simulink model "qbot2_sim_2020a"  (R2020a)
settings: Solver=FixedStepAuto  StartTime=0.0  StopTime=P.t_end  FixedStep=P.dt  RelTol=1e-3
InitFcn:
  | % load_qbot2_sim
StopFcn:
  | if (P.plotsim_flag)
  |     plot_sim(out, P)
  | end
settings Model: Creator=David L Olson  LastModifiedBy=divad

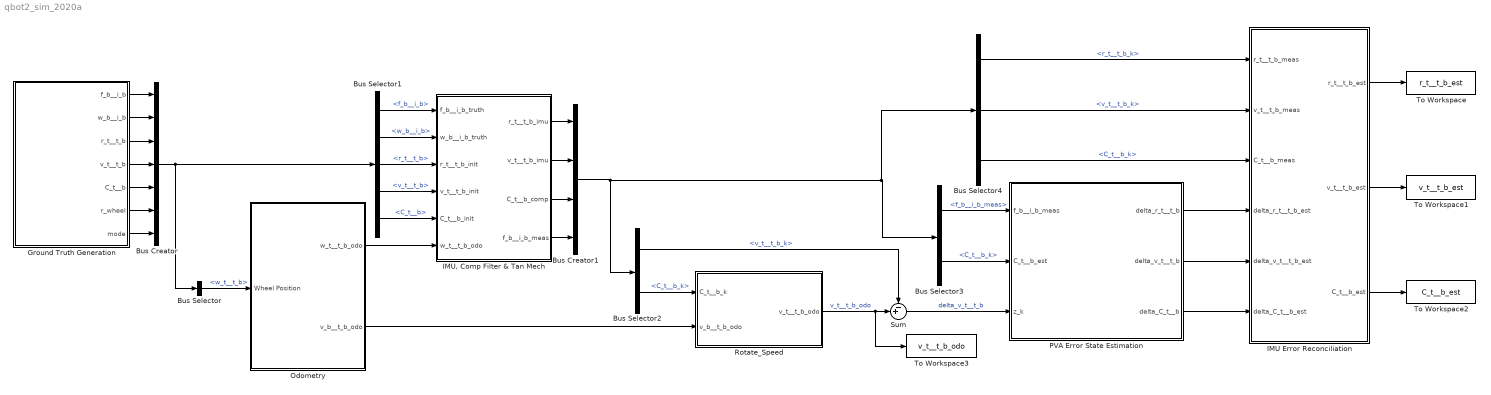
== system qbot2_sim_2020a ==
  Bus Creator : BusCreator  Inputs=7
  Bus Creator1 : BusCreator  Inputs=4
  Bus Selector : BusSelector  OutputSignals=w_t__t_b
  Bus Selector1 : BusSelector  OutputSignals=f_b__i_b,w_b__i_b,r_t__t_b,v_t__t_b,C_t__b
  Bus Selector2 : BusSelector  OutputSignals=v_t__t_b_k,C_t__b_k
  Bus Selector3 : BusSelector  OutputSignals=f_b__i_b_meas,C_t__b_k
  Bus Selector4 : BusSelector  OutputSignals=r_t__t_b_k,v_t__t_b_k,C_t__b_k
  Ground Truth Generation : Subsystem
  IMU Error Reconciliation : MATLAB Function  TreatAsAtomicUnit=on
  "IMU, Comp Filter & Tan Mech" : Subsystem
  Odometry : Subsystem
  PVA Error State Estimation : Subsystem
  Rotate_Speed : MATLAB Function  TreatAsAtomicUnit=on
  Sum : Sum  Inputs=-+|
  To Workspace : ToWorkspace  VariableName=r_t__t_b_est  SampleTime=-1
  To Workspace1 : ToWorkspace  VariableName=v_t__t_b_est  SampleTime=-1
  To Workspace2 : ToWorkspace  VariableName=C_t__b_est  SampleTime=-1
  To Workspace3 : ToWorkspace  VariableName=v_t__t_b_odo  SampleTime=-1
  wires:
  Ground Truth Generation/1(f_b__i_b) -> Bus Creator/1
  Ground Truth Generation/2(w_b__i_b) -> Bus Creator/2
  Ground Truth Generation/3(r_t__t_b) -> Bus Creator/3
  Ground Truth Generation/4(v_t__t_b) -> Bus Creator/4
  Ground Truth Generation/5(C_t__b) -> Bus Creator/5
  Bus Creator/1 -> Bus Selector1/1, Bus Selector/1
  Ground Truth Generation/6(r_wheel) -> Bus Creator/6
  Ground Truth Generation/7(mode) -> Bus Creator/7
  Bus Selector/1 -> Odometry/1(Wheel Position)  "<w_t__t_b>"
  Bus Selector1/1 -> "IMU, Comp Filter & Tan Mech"/1(f_b__i_b_truth)  "<f_b__i_b>"
  Bus Selector1/2 -> "IMU, Comp Filter & Tan Mech"/2(w_b__i_b_truth)  "<w_b__i_b>"
  Bus Selector1/3 -> "IMU, Comp Filter & Tan Mech"/3(r_t__t_b_init)  "<r_t__t_b>"
  Bus Selector1/4 -> "IMU, Comp Filter & Tan Mech"/4(v_t__t_b_init)  "<v_t__t_b>"
  Bus Selector1/5 -> "IMU, Comp Filter & Tan Mech"/5(C_t__b_init)  "<C_t__b>"
  Sum/1 -> PVA Error State Estimation/3(z_k)  "delta_v_t__t_b"
  Odometry/1(w_t__t_b_odo) -> "IMU, Comp Filter & Tan Mech"/6(w_t__t_b_odo)
  Odometry/2(v_b__t_b_odo) -> Rotate_Speed/2(v_b__t_b_odo)
  Rotate_Speed/1(v_t__t_b_odo) -> To Workspace3/1, Sum/2  "v_t__t_b_odo"
  "IMU, Comp Filter & Tan Mech"/1(r_t__t_b_imu) -> Bus Creator1/1
  "IMU, Comp Filter & Tan Mech"/2(v_t__t_b_imu) -> Bus Creator1/2
  "IMU, Comp Filter & Tan Mech"/3(C_t__b_comp) -> Bus Creator1/3
  "IMU, Comp Filter & Tan Mech"/4(f_b__i_b_meas) -> Bus Creator1/4
  Bus Creator1/1 -> Bus Selector4/1, Bus Selector3/1, Bus Selector2/1
  Bus Selector2/2 -> Rotate_Speed/1(C_t__b_k)  "<C_t__b_k>"
  Bus Selector2/1 -> Sum/1  "<v_t__t_b_k>"
  Bus Selector3/1 -> PVA Error State Estimation/1(f_b__i_b_meas)  "<f_b__i_b_meas>"
  Bus Selector3/2 -> PVA Error State Estimation/2(C_t__b_est)  "<C_t__b_k>"
  PVA Error State Estimation/1(delta_r_t__t_b) -> IMU Error Reconciliation/4(delta_r_t__t_b_est)
  PVA Error State Estimation/2(delta_v_t__t_b) -> IMU Error Reconciliation/5(delta_v_t__t_b_est)
  PVA Error State Estimation/3(delta_C_t__b) -> IMU Error Reconciliation/6(delta_C_t__b_est)
  Bus Selector4/1 -> IMU Error Reconciliation/1(r_t__t_b_meas)  "<r_t__t_b_k>"
  Bus Selector4/2 -> IMU Error Reconciliation/2(v_t__t_b_meas)  "<v_t__t_b_k>"
  Bus Selector4/3 -> IMU Error Reconciliation/3(C_t__b_meas)  "<C_t__b_k>"
  IMU Error Reconciliation/1(r_t__t_b_est) -> To Workspace/1
  IMU Error Reconciliation/3(C_t__b_est) -> To Workspace2/1
  IMU Error Reconciliation/2(v_t__t_b_est) -> To Workspace1/1

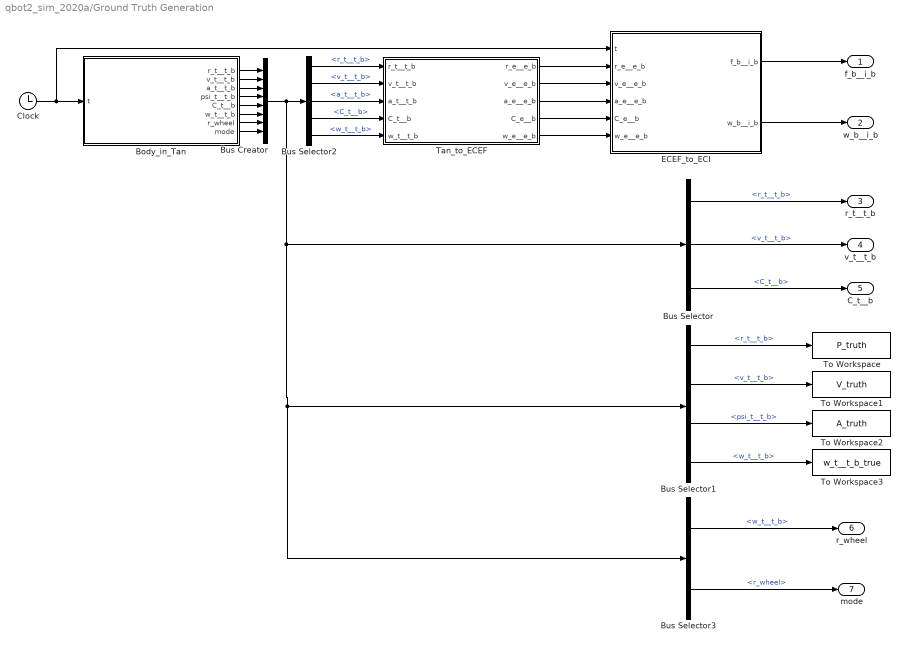
== system qbot2_sim_2020a/Ground Truth Generation ==
  Body_in_Tan : MATLAB Function  TreatAsAtomicUnit=on
  Bus Creator : BusCreator  Inputs=8
  Bus Selector : BusSelector  OutputSignals=r_t__t_b,v_t__t_b,C_t__b
  Bus Selector1 : BusSelector  OutputSignals=r_t__t_b,v_t__t_b,psi_t__t_b,w_t__t_b
  Bus Selector2 : BusSelector  OutputSignals=r_t__t_b,v_t__t_b,a_t__t_b,C_t__b,w_t__t_b
  Bus Selector3 : BusSelector  OutputSignals=w_t__t_b,r_wheel
  Clock : Clock
  ECEF_to_ECI : MATLAB Function  TreatAsAtomicUnit=on
  Tan_to_ECEF : MATLAB Function  TreatAsAtomicUnit=on
  To Workspace : ToWorkspace  VariableName=P_truth  SampleTime=-1
  To Workspace1 : ToWorkspace  VariableName=V_truth  SampleTime=-1
  To Workspace2 : ToWorkspace  VariableName=A_truth  SampleTime=-1
  To Workspace3 : ToWorkspace  VariableName=w_t__t_b_true  SampleTime=-1
  f_b__i_b : Outport
  w_b__i_b : Outport  Port=2
  r_t__t_b : Outport  Port=3
  v_t__t_b : Outport  Port=4
  C_t__b : Outport  Port=5
  r_wheel : Outport  Port=6
  mode : Outport  Port=7
  wires:
  Clock/1 -> Body_in_Tan/1(t), ECEF_to_ECI/1(t)
  Tan_to_ECEF/1(r_e__e_b) -> ECEF_to_ECI/2(r_e__e_b)
  Tan_to_ECEF/3(a_e__e_b) -> ECEF_to_ECI/4(a_e__e_b)
  Tan_to_ECEF/2(v_e__e_b) -> ECEF_to_ECI/3(v_e__e_b)
  Tan_to_ECEF/4(C_e__b) -> ECEF_to_ECI/5(C_e__b)
  Tan_to_ECEF/5(w_e__e_b) -> ECEF_to_ECI/6(w_e__e_b)
  ECEF_to_ECI/2(w_b__i_b) -> w_b__i_b/1
  ECEF_to_ECI/1(f_b__i_b) -> f_b__i_b/1
  Bus Selector/1 -> r_t__t_b/1  "<r_t__t_b>"
  Bus Selector/2 -> v_t__t_b/1  "<v_t__t_b>"
  Bus Selector/3 -> C_t__b/1  "<C_t__b>"
  Bus Selector2/5 -> Tan_to_ECEF/5(w_t__t_b)  "<w_t__t_b>"
  Bus Selector2/4 -> Tan_to_ECEF/4(C_t__b)  "<C_t__b>"
  Bus Selector2/3 -> Tan_to_ECEF/3(a_t__t_b)  "<a_t__t_b>"
  Bus Selector2/2 -> Tan_to_ECEF/2(v_t__t_b)  "<v_t__t_b>"
  Bus Selector2/1 -> Tan_to_ECEF/1(r_t__t_b)  "<r_t__t_b>"
  Bus Selector1/2 -> To Workspace1/1  "<v_t__t_b>"
  Bus Selector1/1 -> To Workspace/1  "<r_t__t_b>"
  Bus Selector1/3 -> To Workspace2/1  "<psi_t__t_b>"
  Bus Creator/1 -> Bus Selector/1, Bus Selector3/1, Bus Selector1/1, Bus Selector2/1
  Bus Selector3/1 -> r_wheel/1  "<w_t__t_b>"
  Bus Selector3/2 -> mode/1  "<r_wheel>"
  Body_in_Tan/1(r_t__t_b) -> Bus Creator/1
  Body_in_Tan/2(v_t__t_b) -> Bus Creator/2
  Body_in_Tan/3(a_t__t_b) -> Bus Creator/3
  Body_in_Tan/4(psi_t__t_b) -> Bus Creator/4
  Body_in_Tan/5(C_t__b) -> Bus Creator/5
  Body_in_Tan/6(w_t__t_b) -> Bus Creator/6
  Body_in_Tan/7(r_wheel) -> Bus Creator/7
  Body_in_Tan/8(mode) -> Bus Creator/8
  Bus Selector1/4 -> To Workspace3/1  "<w_t__t_b>"

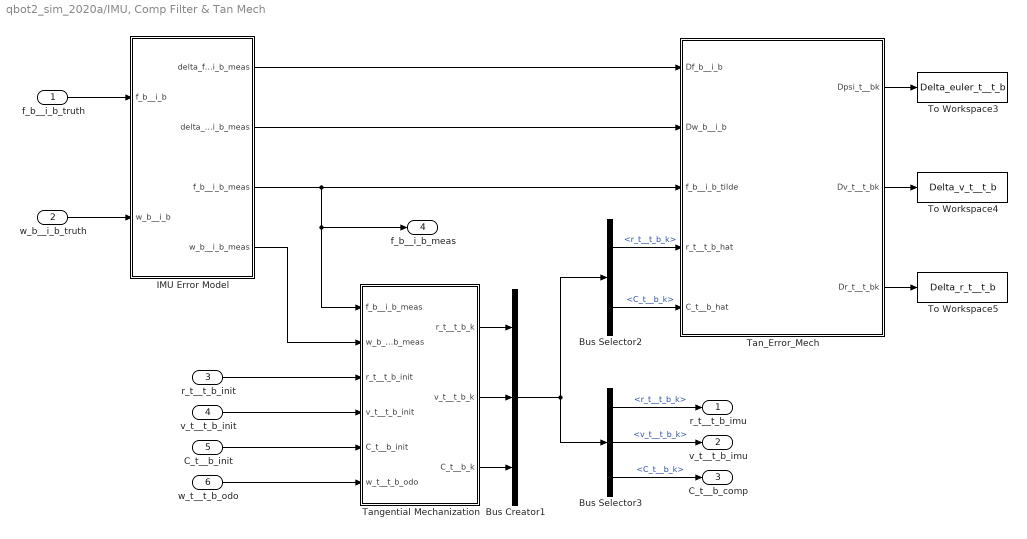
== system qbot2_sim_2020a/IMU, Comp Filter & Tan Mech ==
  f_b__i_b_truth : Inport
  w_b__i_b_truth : Inport  Port=2
  r_t__t_b_init : Inport  Port=3
  v_t__t_b_init : Inport  Port=4
  C_t__b_init : Inport  Port=5
  w_t__t_b_odo : Inport  Port=6
  Bus Creator1 : BusCreator  Inputs=3
  Bus Selector2 : BusSelector  OutputSignals=r_t__t_b_k,C_t__b_k
  Bus Selector3 : BusSelector  OutputSignals=r_t__t_b_k,v_t__t_b_k,C_t__b_k
  IMU Error Model : Subsystem
  Tan_Error_Mech : MATLAB Function  TreatAsAtomicUnit=on
  Tangential Mechanization : Subsystem
  To Workspace3 : ToWorkspace  VariableName=Delta_euler_t__t_b  SampleTime=-1
  To Workspace4 : ToWorkspace  VariableName=Delta_v_t__t_b  SampleTime=-1
  To Workspace5 : ToWorkspace  VariableName=Delta_r_t__t_b  SampleTime=-1
  r_t__t_b_imu : Outport
  v_t__t_b_imu : Outport  Port=2
  C_t__b_comp : Outport  Port=3
  f_b__i_b_meas : Outport  Port=4
  wires:
  f_b__i_b_truth/1 -> IMU Error Model/1(f_b__i_b)
  IMU Error Model/4(w_b__i_b_meas) -> Tangential Mechanization/2(w_b__i_b_meas)
  Tangential Mechanization/3(C_t__b_k) -> Bus Creator1/3
  IMU Error Model/1(delta_f_b__i_b_meas) -> Tan_Error_Mech/1(Df_b__i_b)
  IMU Error Model/3(f_b__i_b_meas) -> Tangential Mechanization/1(f_b__i_b_meas), f_b__i_b_meas/1, Tan_Error_Mech/3(f_b__i_b_tilde)
  w_b__i_b_truth/1 -> IMU Error Model/2(w_b__i_b)
  Tangential Mechanization/2(v_t__t_b_k) -> Bus Creator1/2
  IMU Error Model/2(delta_w_b__i_b_meas) -> Tan_Error_Mech/2(Dw_b__i_b)
  Tangential Mechanization/1(r_t__t_b_k) -> Bus Creator1/1
  Bus Selector2/2 -> Tan_Error_Mech/5(C_t__b_hat)  "<C_t__b_k>"
  C_t__b_init/1 -> Tangential Mechanization/5(C_t__b_init)
  v_t__t_b_init/1 -> Tangential Mechanization/4(v_t__t_b_init)
  Bus Creator1/1 -> Bus Selector2/1, Bus Selector3/1
  Bus Selector3/2 -> v_t__t_b_imu/1  "<v_t__t_b_k>"
  Bus Selector2/1 -> Tan_Error_Mech/4(r_t__t_b_hat)  "<r_t__t_b_k>"
  Bus Selector3/1 -> r_t__t_b_imu/1  "<r_t__t_b_k>"
  r_t__t_b_init/1 -> Tangential Mechanization/3(r_t__t_b_init)
  Tan_Error_Mech/3(Dr_t__t_bk) -> To Workspace5/1
  Tan_Error_Mech/1(Dpsi_t__bk) -> To Workspace3/1
  Tan_Error_Mech/2(Dv_t__t_bk) -> To Workspace4/1
  w_t__t_b_odo/1 -> Tangential Mechanization/6("w_t__t_b_odo ")
  Bus Selector3/3 -> C_t__b_comp/1  "<C_t__b_k>"

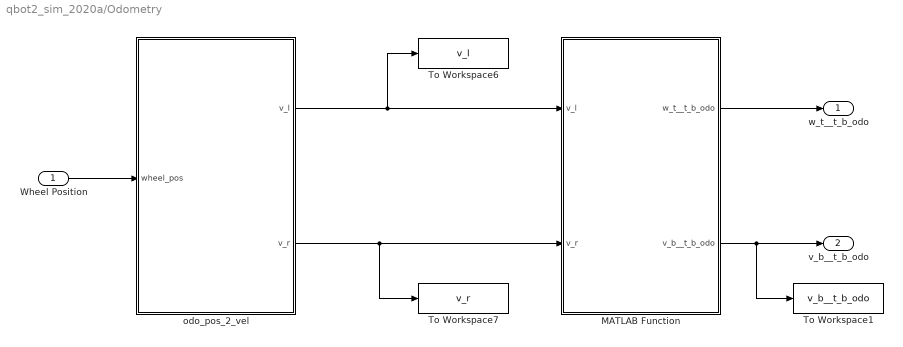
== system qbot2_sim_2020a/Odometry ==
  Wheel Position : Inport
  MATLAB Function : MATLAB Function  TreatAsAtomicUnit=on
  To Workspace1 : ToWorkspace  VariableName=v_b__t_b_odo  SampleTime=-1
  To Workspace6 : ToWorkspace  VariableName=v_l  SampleTime=-1
  To Workspace7 : ToWorkspace  VariableName=v_r  SampleTime=-1
  odo_pos_2_vel : MATLAB Function  TreatAsAtomicUnit=on
  w_t__t_b_odo : Outport
  v_b__t_b_odo : Outport  Port=2
  wires:
  Wheel Position/1 -> odo_pos_2_vel/1(wheel_pos)
  MATLAB Function/1(w_t__t_b_odo) -> w_t__t_b_odo/1
  odo_pos_2_vel/1(v_l) -> To Workspace6/1, MATLAB Function/1(v_l)
  odo_pos_2_vel/2(v_r) -> To Workspace7/1, MATLAB Function/2(v_r)
  MATLAB Function/2(v_b__t_b_odo) -> To Workspace1/1, v_b__t_b_odo/1

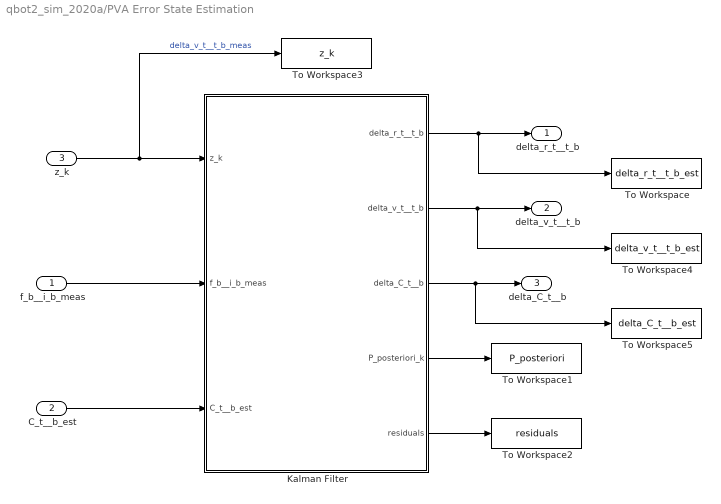
== system qbot2_sim_2020a/PVA Error State Estimation ==
  f_b__i_b_meas : Inport
  C_t__b_est : Inport  Port=2
  z_k : Inport  Port=3
  Kalman Filter : MATLAB Function  TreatAsAtomicUnit=on
  To Workspace : ToWorkspace  VariableName=delta_r_t__t_b_est  SampleTime=-1
  To Workspace1 : ToWorkspace  VariableName=P_posteriori  SampleTime=-1
  To Workspace2 : ToWorkspace  VariableName=residuals  SampleTime=-1
  To Workspace3 : ToWorkspace  VariableName=z_k  SampleTime=-1
  To Workspace4 : ToWorkspace  VariableName=delta_v_t__t_b_est  SampleTime=-1
  To Workspace5 : ToWorkspace  VariableName=delta_C_t__b_est  SampleTime=-1
  delta_r_t__t_b : Outport
  delta_v_t__t_b : Outport  Port=2
  delta_C_t__b : Outport  Port=3
  wires:
  Kalman Filter/4(P_posteriori_k) -> To Workspace1/1
  f_b__i_b_meas/1 -> Kalman Filter/2(f_b__i_b_meas)
  C_t__b_est/1 -> Kalman Filter/3(C_t__b_est)
  Kalman Filter/5(residuals) -> To Workspace2/1
  z_k/1 -> To Workspace3/1, Kalman Filter/1(z_k)  "delta_v_t__t_b_meas"
  Kalman Filter/1(delta_r_t__t_b) -> To Workspace/1, delta_r_t__t_b/1
  Kalman Filter/2(delta_v_t__t_b) -> To Workspace4/1, delta_v_t__t_b/1
  Kalman Filter/3(delta_C_t__b) -> To Workspace5/1, delta_C_t__b/1

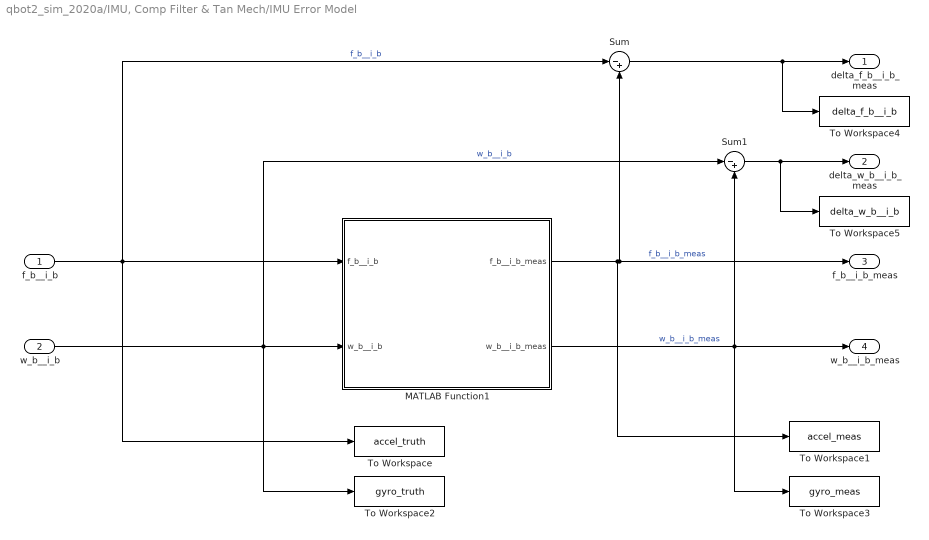
== system qbot2_sim_2020a/IMU, Comp Filter & Tan Mech/IMU Error Model ==
  f_b__i_b : Inport
  w_b__i_b : Inport  Port=2
  MATLAB Function1 : MATLAB Function  TreatAsAtomicUnit=on
  Sum : Sum  Inputs=|-+
  Sum1 : Sum  Inputs=|-+
  To Workspace : ToWorkspace  VariableName=accel_truth  SampleTime=-1
  To Workspace1 : ToWorkspace  VariableName=accel_meas  SampleTime=-1
  To Workspace2 : ToWorkspace  VariableName=gyro_truth  SampleTime=-1
  To Workspace3 : ToWorkspace  VariableName=gyro_meas  SampleTime=-1
  To Workspace4 : ToWorkspace  VariableName=delta_f_b__i_b  SampleTime=-1
  To Workspace5 : ToWorkspace  VariableName=delta_w_b__i_b  SampleTime=-1
  delta_f_b__i_b_meas : Outport
  delta_w_b__i_b_meas : Outport  Port=2
  f_b__i_b_meas : Outport  Port=3
  w_b__i_b_meas : Outport  Port=4
  wires:
  f_b__i_b/1 -> To Workspace/1, Sum/1, MATLAB Function1/1(f_b__i_b)  "f_b__i_b"
  w_b__i_b/1 -> Sum1/1, To Workspace2/1, MATLAB Function1/2(w_b__i_b)  "w_b__i_b"
  MATLAB Function1/1(f_b__i_b_meas) -> f_b__i_b_meas/1, Sum/2, To Workspace1/1  "f_b__i_b_meas"
  MATLAB Function1/2(w_b__i_b_meas) -> Sum1/2, w_b__i_b_meas/1, To Workspace3/1  "w_b__i_b_meas"
  Sum1/1 -> To Workspace5/1, delta_w_b__i_b_meas/1
  Sum/1 -> To Workspace4/1, delta_f_b__i_b_meas/1

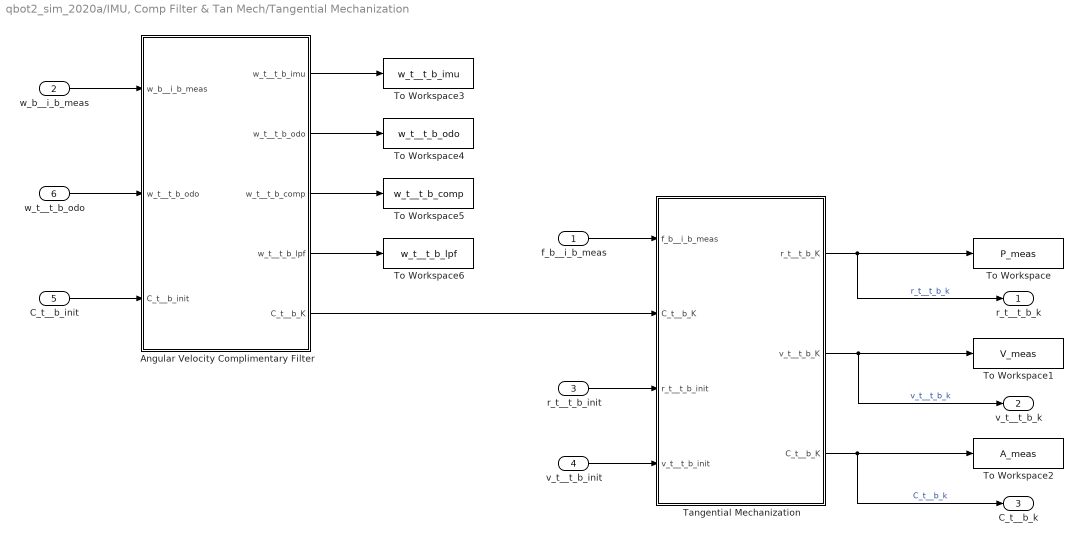
== system qbot2_sim_2020a/IMU, Comp Filter & Tan Mech/Tangential Mechanization ==
  f_b__i_b_meas : Inport
  w_b__i_b_meas : Inport  Port=2
  r_t__t_b_init : Inport  Port=3
  v_t__t_b_init : Inport  Port=4
  C_t__b_init : Inport  Port=5
  "w_t__t_b_odo " : Inport  Port=6
  Angular Velocity Complimentary Filter : MATLAB Function  TreatAsAtomicUnit=on
  Tangential Mechanization : MATLAB Function  TreatAsAtomicUnit=on
  To Workspace : ToWorkspace  VariableName=P_meas  SampleTime=-1
  To Workspace1 : ToWorkspace  VariableName=V_meas  SampleTime=-1
  To Workspace2 : ToWorkspace  VariableName=A_meas  SampleTime=-1
  To Workspace3 : ToWorkspace  VariableName=w_t__t_b_imu  SampleTime=-1
  To Workspace4 : ToWorkspace  VariableName=w_t__t_b_odo  SampleTime=-1
  To Workspace5 : ToWorkspace  VariableName=w_t__t_b_comp  SampleTime=-1
  To Workspace6 : ToWorkspace  VariableName=w_t__t_b_lpf  SampleTime=-1
  r_t__t_b_k : Outport
  v_t__t_b_k : Outport  Port=2
  C_t__b_k : Outport  Port=3
  wires:
  Tangential Mechanization/3(C_t__b_K) -> C_t__b_k/1, To Workspace2/1  "C_t__b_k"
  Tangential Mechanization/1(r_t__t_b_K) -> r_t__t_b_k/1, To Workspace/1  "r_t__t_b_k"
  Tangential Mechanization/2(v_t__t_b_K) -> v_t__t_b_k/1, To Workspace1/1  "v_t__t_b_k"
  f_b__i_b_meas/1 -> Tangential Mechanization/1(f_b__i_b_meas)
  r_t__t_b_init/1 -> Tangential Mechanization/3(r_t__t_b_init)
  v_t__t_b_init/1 -> Tangential Mechanization/4(v_t__t_b_init)
  w_b__i_b_meas/1 -> Angular Velocity Complimentary Filter/1(w_b__i_b_meas)
  C_t__b_init/1 -> Angular Velocity Complimentary Filter/3(C_t__b_init)
  "w_t__t_b_odo "/1 -> Angular Velocity Complimentary Filter/2("w_t__t_b_odo ")
  Angular Velocity Complimentary Filter/5(C_t__b_K) -> Tangential Mechanization/2("C_t__b_K ")
  Angular Velocity Complimentary Filter/1(w_t__t_b_imu) -> To Workspace3/1
  Angular Velocity Complimentary Filter/2(w_t__t_b_odo) -> To Workspace4/1
  Angular Velocity Complimentary Filter/3(w_t__t_b_comp) -> To Workspace5/1
  Angular Velocity Complimentary Filter/4(w_t__t_b_lpf) -> To Workspace6/1

== matlab function qbot2_sim_2020a/IMU Error Reconciliation ==
  data: r_t__t_b_meas input; r_t__t_b_est output; v_t__t_b_meas input; C_t__b_meas input; v_t__t_b_est output; C_t__b_est output; delta_r_t__t_b_est input; delta_v_t__t_b_est input; delta_C_t__b_est input
function [r_t__t_b_est, v_t__t_b_est, C_t__b_est] = ...
    imu_error_reconcile(r_t__t_b_meas, v_t__t_b_meas, C_t__b_meas, ...
                        delta_r_t__t_b_est, delta_v_t__t_b_est, delta_C_t__b_est)

% Reconclie Position
r_t__t_b_est = r_t__t_b_meas - delta_r_t__t_b_est;

% Reconcile Velocity
v_t__t_b_est = v_t__t_b_meas - delta_v_t__t_b_est;

% Reconclie Attitude
C_t__b_est = C_t__b_meas * delta_C_t__b_est;

== matlab function qbot2_sim_2020a/PVA Error State Estimation/Kalman Filter ==
  data: delta_r_t__t_b output; delta_v_t__t_b output; delta_C_t__b output; z_k input; f_b__i_b_meas input; C_t__b_est input; P parameter; P_posteriori_k output; residuals output
function [delta_r_t__t_b, delta_v_t__t_b, delta_C_t__b, P_posteriori_k, residuals] = ...
              IMU_Error_State_Estimation(z_k, f_b__i_b_meas, C_t__b_est, P)
%% IMU Error State Estimation Function
% Recieves error measurements from the difference between odometry and the
% IMU, and provides estimates of that error.  

persistent x_posteriori_k_1 P_posteriori_k_1 A Q_bar 

dt = P.dt;

% Normalize C_t__b_est
C_t__b_est = q2dcm(dcm2q(C_t__b_est));

%% Kalman Filter Prediction Steps

%**************************************************************************
% For first instance only
if (isempty(x_posteriori_k_1))
    
% Set Initial Values for x and P___________________________________________
    x_0 = zeros(15,1);
    P_0 = diag(1000 * [P.gyro.sigma_ARW.^2; ...
                      P.accel.sigma_VRW.^2; ...
                     (P.accel.sigma_VRW * dt).^2; ...
                      P.accel.BI.sigma_n.^2; ...
                      P.gyro.BI.sigma_n.^2]);
    x_posteriori_k_1 = zeros(15,1);
    P_posteriori_k_1 = eye(15);
    
% Build the Contiuous Time Model___________________________________________
    A = zeros(15, 15);
    
    % Values that vary with time
    f_b__i_b_est = f_b__i_b_meas;
    
    % Compute A - Fifth Row
    A(13:15, 13:15) = -eye(3) ./ P.gyro.BI.correlation_time;
    
    % Compute A - Fourth Row
    A(10:12, 10:12) = -eye(3) ./ P.accel.BI.correlation_time;
    
    % Compute A - Third Row
    A(7:9, 4:6) = eye(3);
    
    % Compute A - Second Row
    A(4:6, 1:3) = -vec2ss(C_t__b_est * f_b__i_b_est);
    A(4:6, 4:6) = -2 .* P.Ohm_t__i_e;
    A(4:6, 10:12) = -C_t__b_est;

    % Compute the monstrosity A(4:6, 7:9) a.k.a. A_23
    r_e__e_b_hat = P.r_e__e_t; % initial position is always the origin
    [L_b_hat, ~, ~] = xyz2llh(r_e__e_b_hat, P);
    g_0 = Somigliana(L_b_hat, P);
    r_e__e_S = Geo_Radius(L_b_hat, P);
    A(4:6, 7:9) = P.C_e__t' * ((2 * g_0 * r_e__e_b_hat) / (r_e__e_S * norm(r_e__e_b_hat)^2)) * r_e__e_b_hat' * P.C_e__t;
    
    % Compute A - First Row
    A(1:3, 1:3) = -P.Ohm_t__i_e;
    A(1:3, 13:15) = -C_t__b_est;
    
% Define Q_bar_____________________________________________________________
    Q_vec = [P.gyro.sigma_ARW.^2;   ...       % Attitude Process Noise rad/s
             P.accel.sigma_VRW.^2;  ...       % Velocity Process Noise m/s
             zeros(3,1);         ...          % Position Process Noise
             P.accel.BI.sigma_n.^2; ...       % Accel Bias Instability Process Noise m/s
             P.gyro.BI.sigma_n.^2];           % Gyro  Bias Instability Process Noise rad/s
     
    % Allow for a margin of error for tuning     
    Q_fudge_factor = 1;
    
    % Set Q
    Q_bar = diag(Q_fudge_factor .* Q_vec');
    
% Discritize the Continuous Time Model_____________________________________
    F = eye(15) + A*dt;
    Q = (1/2) * ((F*Q_bar*F') + Q_bar) * dt;
    
% Compute first prediction_________________________________________________
    x_priori_k = F * x_0;
    P_priori_k = (F * P_0 * F') + Q;
    
%**************************************************************************
% All other instances: State Prediction  
else
    
% Re-compute the time varying arguements of A______________________________
    
    % Values that vary with time
    f_b__i_b_est = f_b__i_b_meas;

    % Compute A - Second Row
    A(4:6, 1:3) = -vec2ss(C_t__b_est * f_b__i_b_est);
    A(4:6, 10:12) = -C_t__b_est;
    
    % Compute A - First Row
    A(1:3, 13:15) = -C_t__b_est;
    
% Discritize the Continuous Time Model_____________________________________
    F = eye(15) + A*dt;
    Q = (1/2) * ((F*Q_bar*F') + Q_bar) * dt;
    
    % Compute prediction step
    x_priori_k = (F * x_posteriori_k_1);
    P_priori_k = (F * P_posteriori_k_1 * F') + Q;
    
    % Symmetrisize P
    P_priori_k = (P_priori_k + P_priori_k') / 2;
    
end

%% Kalman Filter Measurement Update Steps
%**************************************************************************

% Set H Matrix - Velocity Aiding Only
H = [vec2ss(x_priori_k(4:6)), eye(3), zeros(3,9)]; % H = [(v_t__t_b,x), I_3, 0_3]

% Build R for odometry
var_v_b__t_b = [(P.sigma_odo_d / P.dt)^2; ...  % Variance of Speed in {b} frame
                 0.005^2; ...                  % Assumed Variance of body frame {y} vel, Nonholomonic Constraints
                 0.005^2];                     % Assumed Variance of body frame {z} vel, Nonholomonic Constraints

% Rotate Noise in {b} frame into the {t} frame
R_vec = C_t__b_est * var_v_b__t_b;

% Allow for Margin of Error
R_fudge_factor = 1.5;

% Set R
R = diag(R_fudge_factor .* R_vec);

% Kalman Gain Computation
K = (P_priori_k * H') / (H * P_priori_k * H' + R);

% compute residuals
residuals = z_k - H*x_priori_k;

% A Posteriori State and Covariance Update
x_posteriori_k = x_priori_k + K*(z_k - H*x_priori_k);
P_posteriori_k = (eye(15) - K*H) * P_priori_k;

%Symmetrisize P
P_posteriori_k = (P_posteriori_k + P_posteriori_k') / 2;

%% Pick-off State Estimates for Function Output

% State Estimates (AVP -> PVA)
delta_x_t__t_b_est = ...
           [x_posteriori_k(7:9); x_posteriori_k(4:6); x_posteriori_k(1:3)];

% Pull Off Position, Velocity, and Attitude Error Separately
delta_r_t__t_b = delta_x_t__t_b_est(1:3);
delta_v_t__t_b = delta_x_t__t_b_est(4:6);
delta_k_t__t_b = delta_x_t__t_b_est(7:9);

% Create and Normalize delta_C_t__b
delta_C_t__b = k2dcm(delta_k_t__t_b);
delta_C_t__b = q2dcm(dcm2q(delta_C_t__b));
       
%% Save State Estimates for Next Loop

x_posteriori_k_1 = x_posteriori_k;
P_posteriori_k_1 = P_posteriori_k;

end

== matlab function qbot2_sim_2020a/Odometry/odo_pos_2_vel ==
  data: wheel_pos input; v_l output; v_r output; P parameter
%% Odometry True Position to Noisy Wheel Velocities
function [v_l, v_r]= pos2vel(wheel_pos, P)
                                                     
% Initialize Inital Conditions
persistent d_l_k_1 d_r_k_1

if (isempty(d_l_k_1))
    d_l_k_1 = 0;
    d_r_k_1 = 0;
end

% ISolate current wheel positions
d_l_k = wheel_pos(1,:);
d_r_k = wheel_pos(2,:);

% Build randn quantities from etrinsic functions
coder.extrinsic('randn');

% Preallocate Memory
randn1 = 0;
randn2 = 0;

% Build the randn variables
randn1 = randn;
randn2 = randn;

% Add Noise to Measurements if desired
if (P.odo_error_flag == true)
    d_l_k = d_l_k + P.sigma_odo_d * randn1;
    d_r_k = d_r_k + P.sigma_odo_d * randn2;
end

% Take this psuedo non-casual derivative
v_l = (d_l_k - d_l_k_1) / P.dt;
v_r = (d_r_k - d_r_k_1) / P.dt;

% Set the Current Values as the Previous Values
d_l_k_1 = d_l_k;
d_r_k_1 = d_r_k;

== matlab function qbot2_sim_2020a/IMU, Comp Filter & Tan Mech/Tangential Mechanization/Angular Velocity Complimentary Filter ==
  data: w_b__i_b_meas input; w_t__t_b_imu output; w_t__t_b_odo input; C_t__b_init input; w_t__t_b_odo output; w_t__t_b_comp output; w_t__t_b_lpf output; C_t__b_K output; P parameter
function [w_t__t_b_imu, w_t__t_b_odo, w_t__t_b_comp, w_t__t_b_lpf, C_t__b_K] = ...
          complimentary_filter(w_b__i_b_meas, w_t__t_b_odo, C_t__b_init, P)

% This block implments a complimentary filter between z-gyro measurements
% and odometry angular veocity measurements and then provides a corrected
% version of C_t__b_k

persistent C_t__b_K_1 delta_w_t__t_b_k_1 delta_w_t__t_b_lpf_k_1

% Initialize on First Time Step
if (isempty(C_t__b_K_1))
    
    % Use "truth" to initialize on first time step
    C_t__b_K   = C_t__b_init;
    
    % Store current values as old values for next iteration
    C_t__b_K_1   = C_t__b_K;

    % Set Up Complimentary Filter Values
    delta_w_t__t_b_k_1 = zeros(3,1);
    delta_w_t__t_b_lpf_k_1 = zeros(3,1);
    
    % Return Other Output Values
    w_t__t_b_imu = C_t__b_K_1*w_b__i_b_meas - P.C_e__t'*P.w_i__i_e;
    w_t__t_b_comp = w_t__t_b_imu;
    w_t__t_b_lpf = w_t__t_b_imu;
    
%% For all other time steps
else
    
    % Employ Complimentary Filter__________________________________________
    if (P.use_comp_filter == true)
        
        % Calculate w_t__t_b_imu
        w_t__t_b_imu = C_t__b_K_1*w_b__i_b_meas - P.C_e__t'*P.w_i__i_e;
        
        % Take the differene between the odo and imu measurements
        delta_w_t__t_b = w_t__t_b_odo - w_t__t_b_imu;
        
        % Pass the w error through the Low Pass Filter (LPF)
        w_t__t_b_lpf = -P.lpf_den_1 .* delta_w_t__t_b_lpf_k_1 + ...
                        P.lpf_num_1 .* delta_w_t__t_b + ...
                        P.lpf_num_2 .* delta_w_t__t_b_k_1;
        
        % Sum up the LPF'd error and IMU meas
        w_t__t_b_comp = w_t__t_b_imu + w_t__t_b_lpf;
        
        % Catch for when w_t__t_b is super super small
        if (norm(w_t__t_b_comp) < (5 * eps))
            C_t__b_K = C_t__b_K_1;
        else
            C_t__b_K = Rodrigues_k(w_t__t_b_comp * P.dt) * C_t__b_K_1;
        end
    
    % If not using Complimentary Filter____________________________________
    else
        
        % Calculate w_t__t_b_imu
        w_t__t_b_imu = C_t__b_K_1*w_b__i_b_meas - P.C_e__t'*P.w_i__i_e;
        
        % Catch for when w_t__t_b is super super small
        if (norm(w_t__t_b_imu) < (5 * eps))
            C_t__b_K = C_t__b_K_1;
        else
            C_t__b_K = Rodrigues_k(w_t__t_b_imu * P.dt) * C_t__b_K_1;
        end
        
        % Return zeros for comp filter variables
        w_t__t_b_comp = zeros(3,1);
        w_t__t_b_lpf = zeros(3,1);
        delta_w_t__t_b = zeros(3,1);
        delta_w_t__t_b_k_1 = zeros(3,1);
        delta_w_t__t_b_lpf_k_1 = zeros(3,1);
        
    end
    
    % Normalize C_t__b_K___________________________________________________
    C_t__b_K = q2dcm(dcm2q(C_t__b_K));
    
    
% Store New Value as the Old_______________________________________________
C_t__b_K_1 = C_t__b_K;
delta_w_t__t_b_k_1 = delta_w_t__t_b;
delta_w_t__t_b_lpf_k_1 = w_t__t_b_lpf;

end

== matlab function qbot2_sim_2020a/Rotate_Speed ==
  data: C_t__b_k input; v_t__t_b_odo output; v_b__t_b_odo input
function v_t__t_b_odo = rotate_speed(C_t__b_k, v_b__t_b_odo)

% Rotate Speed in the body frame into the {t} frame
v_t__t_b_odo = C_t__b_k * v_b__t_b_odo;

== matlab function qbot2_sim_2020a/Ground Truth Generation/Body_in_Tan ==
  data: r_t__t_b output; v_t__t_b output; a_t__t_b output; psi_t__t_b output; C_t__b output; w_t__t_b output; t input; P parameter; r_wheel output; mode output
function [r_t__t_b, v_t__t_b, a_t__t_b, psi_t__t_b, C_t__b, w_t__t_b, r_wheel, mode] = ...
                                           Body_in_Tan(t, P)
                                       
%% QBOT2_TAN_GROUND_TRUTH_GEN Generates the motion of the body of the Qbot2
%wrt to the tangential frame.  

% Creating figure eight loop pattern for Qbot2.  The motion is unrealistic
% for the robot itself, however for now this verify all equations have been
% implemented correctly in all 3 dimensions.  

persistent k

% Initialize k on first run
if (isempty(k))
    k = 1;
end

% Pull Motion Plan Values from P structure
r_t__t_b = P.r_t__t_b(:,k);
v_t__t_b = P.v_t__t_b(:,k);
a_t__t_b = P.a_t__t_b(:,k);
psi_t__t_b = [0; 0; P.psi_t__t_b(k)];
C_t__b = rotate_z(psi_t__t_b(3));
w_t__t_b = P.w_t__t_b(:,k);
r_wheel = P.r_wheel(:,k);
mode = P.mode(k);

% Normalize C_t__b
C_t__b = q2dcm(dcm2q(C_t__b));

% Update k
k = k + 1;

end

== matlab function qbot2_sim_2020a/IMU, Comp Filter & Tan Mech/Tangential Mechanization/Tangential Mechanization ==
  data: f_b__i_b_meas input; C_t__b_K input; r_t__t_b_init input; v_t__t_b_init input; r_t__t_b_K output; P parameter; v_t__t_b_K output; C_t__b_K output
function [r_t__t_b_K, v_t__t_b_K, C_t__b_K] = Tan_Mech(f_b__i_b_meas, C_t__b_K, r_t__t_b_init, v_t__t_b_init, P)

%% Tan_Mech
% Provides tangential mechanization for kinematic states position, velocity
% and attitude (PVA).  It does this solely based on accel and gyro
% measurements, which come from the IMU block.  The first time step is
% initialized from the ground truth block.  

persistent r_t__t_b_K_1 v_t__t_b_K_1 g_t__b

% Initialize on First Time Step
if (isempty(r_t__t_b_K_1))
    
    % Use "truth" to initialize on first time step
    r_t__t_b_K = r_t__t_b_init;
    v_t__t_b_K = v_t__t_b_init;
    
    % Store current values as old values for next iteration
    r_t__t_b_K_1 = r_t__t_b_K;
    v_t__t_b_K_1 = v_t__t_b_K;
    
    % Calculate and store the vector g_t__b
    r_e__e_b = P.r_e__e_t + P.C_e__t*r_t__t_b_init;         % Compute r_e__e_b
    [L_b, lambda_b, h_b] = xyz2llh(r_e__e_b, P);            % Compute the lat, lon, and height
    g_n__b = [0; 0; gravity(L_b, h_b, P)];                  % Compute the acceleration due to gravity
    C_e__n = Lat_Lon_2C_e__n(L_b, lambda_b);                % Compute C_e__n
    g_e__b = C_e__n * g_n__b;                               % Compute the gravity of the body in the {e} frame
    g_t__b = P.C_e__t' * g_e__b;                            % Compute the gravity of the body in the {t} frame 
    
% Every Other Time Step____________________________________________________
else
    
    % f_t__i_b Specific Force Update
    f_t__i_b = C_t__b_K * f_b__i_b_meas;
    
    % a_t__t_b Acceleration Vector Update
    
    a_t__t_b = f_t__i_b + g_t__b - 2*P.Ohm_t__i_e*v_t__t_b_K_1;
    
    % v_t__t_b Velocity Vector Update
    v_t__t_b_K = v_t__t_b_K_1 + a_t__t_b*P.dt;
    
    % r_t__t_b Position Vector Update
    r_t__t_b_K = r_t__t_b_K_1 + v_t__t_b_K_1*P.dt + a_t__t_b*((P.dt^2)/2);
    
    % Store new PVA as old PVA
    r_t__t_b_K_1 = r_t__t_b_K;
    v_t__t_b_K_1 = v_t__t_b_K;
    
end

== matlab function qbot2_sim_2020a/Ground Truth Generation/Tan_to_ECEF ==
  data: r_t__t_b input; v_t__t_b input; a_t__t_b input; C_t__b input; w_t__t_b input; r_e__e_b output; v_e__e_b output; a_e__e_b output; C_e__b output; w_e__e_b output; P parameter
function [r_e__e_b, v_e__e_b, a_e__e_b, C_e__b, w_e__e_b] = ...
             Tan_to_ECEF(r_t__t_b, v_t__t_b, a_t__t_b, C_t__b, w_t__t_b, P)
         
%% Tan_to_ECEF 
% Transfroms motion in the {t} frame into the {e} frame.  The 'P' structure
% contains data relevant to making the {t}->{e} transforms specifically to
% my house in Minot ND.  (1124 9th St NW, Minot ND 58703)

% Position of the {b} frame wrt the {e} frame resolved in {e} (m)
r_e__e_b = P.r_e__e_t + P.C_e__t*r_t__t_b;

% Velocity of the {b} frame wrt the {e} frame resolved in {e} (m/s)
v_e__e_b = P.C_e__t*v_t__t_b;
       
% Acceleration of the b-frame wrt the e-frame resolved in {e} (m/s^2)
a_e__e_b = P.C_e__t*a_t__t_b;
        
%Attitude of the {b} frame wrt the {e} frame (unitless)
C_e__b = P.C_e__t*C_t__b;         

% Normalize C_e__b
C_e__b = q2dcm(dcm2q(C_e__b));

% Angular velocity of the {b} frame wrt the {e} frame resolved in {e} (rad/s)
w_e__e_b = P.C_e__t*w_t__t_b;

== matlab function qbot2_sim_2020a/Ground Truth Generation/ECEF_to_ECI ==
  data: t input; f_b__i_b output; r_e__e_b input; v_e__e_b input; a_e__e_b input; C_e__b input; w_e__e_b input; w_b__i_b output; P parameter
function [f_b__i_b, w_b__i_b] = ...
          ECEF_to_ECI(t, r_e__e_b, v_e__e_b, a_e__e_b, C_e__b, w_e__e_b, P)

%% ECEF to ECI
% Transforms motion from the ECEF frame to the ECI frame
% This assumes the simulation always starts at 0000z

% Calculate g_n__b only once, since area of travel is so small
persistent g_e__b

if (isempty(g_e__b))
    [L_b, lambda_b, h_b] = xyz2llh(r_e__e_b, P);
    g_n__b = [0; 0; gravity(L_b, h_b, P)];
    C_e__n = Lat_Lon_2C_e__n(L_b, lambda_b);
    g_e__b = C_e__n * g_n__b;
end

% Generate earth's rotation from {i} frame to {e} frame
theta_ie = P.w_ie * t + 0;

C_i__e = [cos(theta_ie), -sin(theta_ie), 0; ...
          sin(theta_ie),  cos(theta_ie), 0; ...
          0,              0,             1];    
      
% Position of {b} frame wrt {t} frame resolved in {i} frame (m)
r_i__i_b = C_i__e*r_e__e_b;

% Velocity of {b} frame wrt {i} frame resolved in {i} frame (m/s)
v_i__i_b = C_i__e*v_e__e_b + P.Ohm_i__i_e*C_i__e*r_e__e_b;

% Acceleration of {b} frame wrt {i} frame resolved in {i} frame (m/s^2)
a_i__i_b = C_i__e*a_e__e_b + 2*P.Ohm_i__i_e*C_i__e*v_e__e_b + ...
                                 P.Ohm_i__i_e*P.Ohm_i__i_e*C_i__e*r_e__e_b;
                                       
% Attitude of {b} frame wrt to {i} frame
C_i__b = C_i__e*C_e__b;

% Normalize C_i__b
C_i__b = q2dcm(dcm2q(C_i__b));

% Angular Velocity: Ideal Gyro Measurements
w_b__i_b = C_i__b' * (P.w_i__i_e + C_i__e*w_e__e_b);

% Specific Force: Ideal Accel Measurements
f_b__i_b = C_i__b' * (a_i__i_b - C_i__e*g_e__b - ...
                                       P.Ohm_i__i_e*P.Ohm_i__i_e*r_i__i_b);

== matlab function qbot2_sim_2020a/IMU, Comp Filter & Tan Mech/IMU Error Model/MATLAB Function1 ==
  data: f_b__i_b input; f_b__i_b_meas output; w_b__i_b input; w_b__i_b_meas output; P parameter
function [f_b__i_b_meas, w_b__i_b_meas] = IMU(f_b__i_b, w_b__i_b, P)
% IMU models the IMU error characteristics, taking truth as the input and
% outputs measurements that are subject to errors.  These errors stem from
% data obtained from the VN200 used for hardware implementation.  

%% Function Initializatoin

persistent b_g_BI b_a_BI

if isempty(b_g_BI)
    b_g_BI = [0; 0; 0];
    b_a_BI = [0; 0; 0];
end

%% Define P

%  General P
dt = P.dt;
Fs = P.Fs;
I3 = eye(3);

% Gyro Related Terms
b_g_BI_sigma_n = P.gyro.BI.sigma_n;  % Bias - White Noise driving the Bias Instability 1-sigma (rad/s)

tau_g        = P.gyro.BI.correlation_time;  % Correlation time for the bias instability (sec)
b_g_FB       = P.gyro.b_g_FB;               % Bias - Fixed Bias term (rad/s)

sigma_ARW   = P.gyro.sigma_ARW;             % Standard deviation of white noise due to ARW (rad/s)
M_g         = P.gyro.M_g;                   % The combined Gyro Misalignment/Scale-Factor matrix
G_g         = P.gyro.G_g;                   % The gyro G-sensitivity matrix (rad/sec/g)

 % Accel related terms   
b_a_BI_sigma_n = P.accel.BI.sigma_n;        % Bias - White noise driving the Bias Instability 1-sigma (m/s^2)

tau_a        = P.accel.BI.correlation_time; % Correlation time for the bias instability (sec)
b_a_FB       = P.accel.b_a_FB;              % Bias - Fixed Bias term (m/s^2)

sigma_VRW   = P.accel.sigma_VRW;            % Standard deviation of white noise due to VRW (m/s^2)
M_a         = P.accel.M_a;                  % The combined Gyro Misalignment/Scale-Factor matrix    

% Build randn quantities from etrinsic functions
coder.extrinsic('randn');

% Preallocate Memory
randn1 = zeros(3,1);
randn2 = zeros(3,1);
randn3 = zeros(3,1);
randn4 = zeros(3,1);

% Build the randn variables
randn1 = randn(3,1);
randn2 = randn(3,1);
randn3 = randn(3,1);
randn4 = randn(3,1);

%++++++++++++++++++++++++++++++++++++++++++++++++++++++++++++++++++++++++++
% Gyro Model:
%++++++++++++++++++++++++++++++++++++++++++++++++++++++++++++++++++++++++++

% Bias terms
b_g_BS = P.gyro.b_g_BS;                                        % Bias - Bias Stability Bias term (rad/s)
b_g_BI = exp(-dt/tau_g) * b_g_BI + randn1.*b_g_BI_sigma_n; % Bias - Markov Bias Instability Bias term (rad/s)
b_g = b_g_BI + b_g_FB + b_g_BS;                                % All three bias terms (rad/s)

% Noise terms
w_g = sigma_ARW .* randn2;                                 % Gyro noise (rad/sec)

% Including all of the error terms
w_b__i_b_meas = b_g + (I3 + M_g) * w_b__i_b + G_g * f_b__i_b + w_g;

%++++++++++++++++++++++++++++++++++++++++++++++++++++++++++++++++++++++++++
% Accelerometer Model
%++++++++++++++++++++++++++++++++++++++++++++++++++++++++++++++++++++++++++

% Bias terms
b_a_BS = P.accel.b_a_BS;                                       % Bias - Bias Stability Bias term (m/s^2)
b_a_BI = exp(-dt/tau_a) * b_a_BI + randn3.*b_a_BI_sigma_n; % Bias - Markov Bias Instability Bias term (m/s^2)
b_a = b_a_BI + b_a_FB + b_a_BS;                                % All three bias terms (m/s^2)

% Noise terms
w_a = sigma_VRW .* randn4;                                 % Accelerometer noise (in m/s^2)

% Including all of the error terms
f_b__i_b_meas = b_a + (I3 + M_a) * f_b__i_b + w_a;

== matlab function qbot2_sim_2020a/IMU, Comp Filter & Tan Mech/Tan_Error_Mech ==
  data: Df_b__i_b input; Dpsi_t__bk output; Dw_b__i_b input; f_b__i_b_tilde input; r_t__t_b_hat input; C_t__b_hat input; Dv_t__t_bk output; Dr_t__t_bk output; P parameter
function [Dpsi_t__bk, Dv_t__t_bk, Dr_t__t_bk] = Tan_Error_mech(Df_b__i_b, Dw_b__i_b, f_b__i_b_tilde, r_t__t_b_hat, C_t__b_hat, P)
%#codegen
% FUNCTION DESCRIPTION:
%   Implements the Tangential Frame Error-Mechanization
%
% INPUTS:
%   Df_b__i_b       = Error in Current Accel measurements (m/s^2)
%   Dw_b__i_b       = Error in Current gyro measurements (rad/s)
%   f_b__i_b_tilde  = Current Accel measurements (m/s^2)
%   r_t__t_b_hat    = Position estimate from TAN mech (meters)
%   C_t__b_hat      = Attitude estimate from TAN mech
%
% OUTPUTS:
%   Dpsi_t__bk      = Delta psi      vector (rad)
%   Dv_t__t_bk      = Delta velocity vector (meters/sec)
%   Dr_t__t_bk      = Delta position vector (meters)
%
%  Reference:  EE 440 Lecture notes:
%       lectures 29 & 30
%  NOTES:
%    Groves Chap 14 Section 2

persistent Delta_PVAk_1

dt         = P.dt;          % Time step (sec)
I3         = eye(3);                % 3X3 Identity matrix
Ohm_i__i_e = P.Ohm_i__i_e;  % Skew symmetric version of w_i__i_e (rad/s)
C_e__t     = P.C_e__t;   	% Attitude of t-frame wrt e-frame (a constant matrix)
C_t__e     = C_e__t';
r_e__e_t   = P.r_e__e_t;    % Position of org of t-frame wrt e-frame resolved in e-frame
   
if isempty(Delta_PVAk_1)    
    Delta_PVAk_1  = zeros(9,1);     % Initialize Delta_PVA(k-1)
    Delta_PVAk    = zeros(9,1);     % Initialize Delta_PVA(k-1)
else
    Delta_PVAk = eye(9);
%% Build the F matrix: See lecture 29 slide 7
    O3 = zeros(3,3);
% First row:
    Ohm_t__i_e = C_t__e * Ohm_i__i_e * C_e__t;  % Earth rate in the t-frame

% Second row:
    F21 = -vec2ss(C_t__b_hat * f_b__i_b_tilde); % Vector to Skew-Symmetric
  % Now build F23
    r_e__e_b_hat = r_e__e_t + C_e__t * r_t__t_b_hat;
    [L_b_hat, lambda_b_hat, h_b_hat] = xyz2llh(r_e__e_b_hat, P);
    gamma_e__i_b = gamma__i_b(r_e__e_b_hat, P);
    r_e__e_S = Geo_Radius(L_b_hat, P);
 
    F23 = -C_t__e * 2 * gamma_e__i_b * r_e__e_b_hat' / (r_e__e_S * norm(r_e__e_b_hat)) * C_e__t;
     
    F = [ -Ohm_t__i_e   ,  O3               , O3
           F21          , -2* Ohm_t__i_e    , F23
           O3           ,  I3               , O3];

%% Build the B matrix: See lecture 29 slide 7
    B = [O3         , C_t__b_hat
         C_t__b_hat , O3
         O3         , O3];

%% Transform Eqns from continuous-time to discrete-time: Lecture 30 slides 9-10
    Phi = eye(9) + F*dt;                % Estimate of exp(F dt) = I + F dt + F^2 dt^2 /2! + ...
	G  = (eye(9)*dt + F*dt^2/2) * B;    % Estimate of G = A^-1 (exp(F dt) - I ) B = (I dt + F dt^2 /2! + ...) B

    Delta_PVAk = Phi*Delta_PVAk_1 + G * [Df_b__i_b; Dw_b__i_b];

    Delta_PVAk_1 = Delta_PVAk;          % Store Delta_PVA(k) into Delta_PVA(k-1) for next iteration
end

Dk_t__bk = Delta_PVAk(1:3,1);   % Extract the Attitude errror terms
[y, p, r] = dcm2ypr(k2dcm(Dk_t__bk));
Dpsi_t__bk = [r; p; y];
Dv_t__t_bk = Delta_PVAk(4:6,1);   % Extract the velocity errror terms
Dr_t__t_bk = Delta_PVAk(7:9,1);   % Extract the position errror terms
end     % End of function

== matlab function qbot2_sim_2020a/Odometry/MATLAB Function ==
  data: w_t__t_b_odo output; v_l input; v_b__t_b_odo output; v_r input; P parameter
%% Odometry Mechanization
function [w_t__t_b_odo, v_b__t_b_odo]= odo_mech(v_l, v_r, P)
                                                     
% Return Angular Velocity
w_t__t_b_odo = [0; 0; (v_l - v_r)/(2*P.radius)];

% Return Speed
v_b__t_b_odo = [((v_l + v_r)/2); 0; 0];
